simulink model "celBebe"  (R2020a)
settings: Solver=FixedStepAuto  StartTime=0.0  StopTime=10.0  RelTol=1e-3
undefined symbols (not defined in the file): AA, B9, blue, green, red
libraries: androiduilib x4, androidaudiovideolib x3, simulink x2, androidcommunicationlib x1, visionsources x1
settings Model: Creator=luisi  LastModifiedBy=luisi
settings OptimizationCC: EnhancedBackFolding=on  PassReuseOutputArgsAs=Individual arguments  ZeroExternalMemoryAtStartup=off  ZeroInternalMemoryAtStartup=off  MaxStackSize=64  OptimizeBlockOrder=speed  DifferentSizesBufferReuse=on  OptimizationCustomize=off  EfficientTunableParamExpr=on
settings DebuggingCC: ParameterTunabilityLossMsg=error
settings HardwareCC: ProdBitPerPointer=32  ProdBitPerSizeT=32  ProdBitPerPtrDiffT=32  ProdLargestAtomicInteger=Long  ProdLargestAtomicFloat=Double  ProdWordSize=32  ProdHWDeviceType=ARM Compatible->ARM Cortex
settings SFSimCC: MATLABDynamicMemAlloc=off
settings RTWCC: SystemTargetFile=ert.tlc  HardwareBoard=Android Device  TemplateMakefile=ert_default_tmf  RTWVerbose=off  Toolchain=Android SDK/NDK Tools
settings CodeAppCC: ForceParamTrailComments=on  IgnoreCustomStorageClasses=off  OperatorAnnotations=on  SimulinkDataObjDesc=on  SFDataObjDesc=on  InsertBlockDesc=on
settings ERTTargetCC: ExtModeMexArgs='localhost'

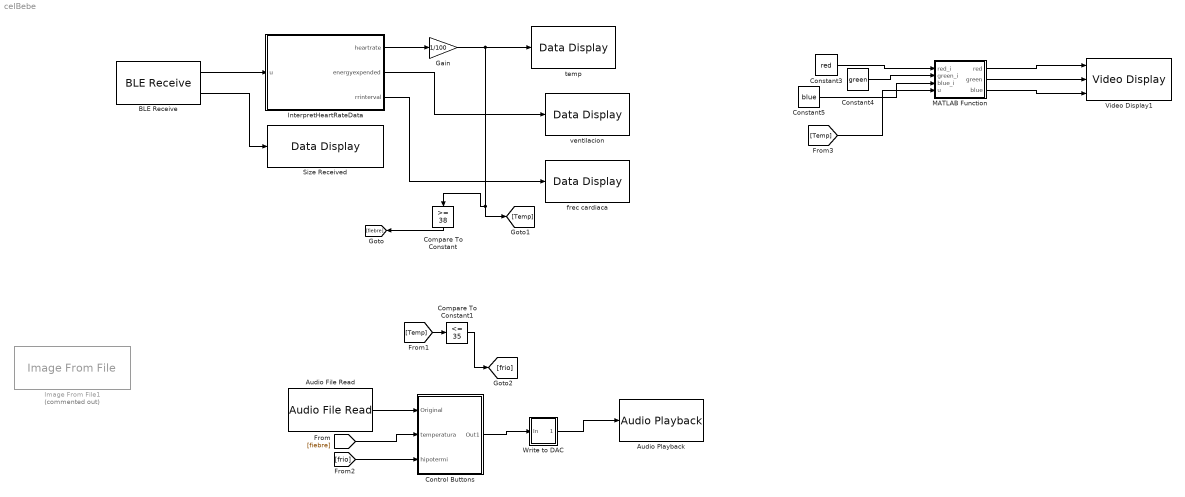
== system celBebe ==
  " BLE Receive" : androidcommunicationlib/BLE Receive  DeviceMode=Central (Client)  BluetoothAddress=4F:B9:1D:3B:34:AA  CharUUID=00002a37-0000-1000-8000-00805f9b34fb  ServiceUUID=0000180d-0000-1000-8000-00805f9b34fb  device=Redmi  character="Heart Rate\\Heart Rate  Measurement"  CustomService=off  ServiceName=Heart Rate  CharacteristicName="Heart Rate  Measurement"  CustomServiceUUID=<Enter Service UUID>  CustomCharUUID=<Enter Characteristic UUID>  DataSize=7  SampleTime=0.1  charseruuid=00001801-0000-1000-8000-00805f9b34fb\00002a05-0000-1000-8000-00805f9b34fb  seruuid=00001810-0000-1000-8000-00805f9b34fb  PeripheralService=0000180d-0000-1000-8000-00805f9b34fb  PeripheralCharacteristic=00002a37-0000-1000-8000-00805f9b34fb  chruuid=00002a37-0000-1000-8000-00805f9b34fb  BLEId=celBebe/_BLE_Receive  Devicename=Redmi  IsCustomService=0
      settings: SourceProductBaseCode=ANDROID
  Audio File Read : androidaudiovideolib/Audio File Read  FileName=C:\Users\luisi\Downloads\baby.mp3  FrameSize=4410
      settings: SourceProductBaseCode=ANDROID
  Audio Playback : androidaudiovideolib/Audio Playback  SampleFreq=44100  AudioSamplingFreq=44100  SampleTime=0.1  DeviceStr=0  QueueDuration=0  BlockPlatform=Android
      settings: SourceProductBaseCode=ANDROID
  Compare To Constant : simulink/Logic and Bit Operations/Compare To Constant  relop=>=  const=38  OutDataTypeStr=boolean
  Compare To Constant1 : simulink/Logic and Bit Operations/Compare To Constant  relop=<=  const=35  OutDataTypeStr=boolean
  Constant3 : Constant  Value=red
  Constant4 : Constant  Value=green
  Constant5 : Constant  Value=blue
  Control Buttons : Subsystem
  Gain : Gain  Gain=1/100
  Image From File1 : visionsources/Image From File  Tag=vipblks_nd  Commented=on  FileName=C:\Users\luisi\Downloads\victoria.jpg  Ts=inf  imagePorts=Separate color signals  OutPortLabels=R|G|B  ImageDataType=uint8  sdImageDataType=uint(8)  Signed=on  WordLength=16  FractionLengthMode=User-defined  FractionLength=15
  InterpretHeartRateData : MATLAB Function  TreatAsAtomicUnit=on
  MATLAB Function : MATLAB Function  TreatAsAtomicUnit=on
  Size Received : androiduilib/Data Display  DataDisplayId=celBebe/Size_Received  Format=Float  Precision=6  SimulateUsing=Code generation  blockPlatform=Android
      settings: SourceProductBaseCode=ANDROID
  Video Display1 : androidaudiovideolib/Video Display  BlockPlatform=Android
      settings: SourceProductBaseCode=ANDROID
  Write to DAC : Subsystem
  frec cardiaca : androiduilib/Data Display  DataDisplayId=celBebe/frec_cardiaca  Format=Integer  Precision=6  SimulateUsing=Code generation  blockPlatform=Android
      settings: SourceProductBaseCode=ANDROID
  temp : androiduilib/Data Display  DataDisplayId=celBebe/temp  Format=Float  Precision=2  SimulateUsing=Code generation  blockPlatform=Android
      settings: SourceProductBaseCode=ANDROID
  ventilacion : androiduilib/Data Display  DataDisplayId=celBebe/ventilacion  Format=Integer  Precision=6  SimulateUsing=Code generation  blockPlatform=Android
      settings: SourceProductBaseCode=ANDROID
  wires:
  " BLE Receive"/2 -> Size Received/1
  " BLE Receive"/1 -> InterpretHeartRateData/1(u)
  Compare To Constant/1 -> [fiebre]
  InterpretHeartRateData/1(heartrate) -> Gain/1
  InterpretHeartRateData/2(energyexpended) -> ventilacion/1
  InterpretHeartRateData/3(rrinterval) -> frec cardiaca/1
  Audio File Read/1 -> Control Buttons/1(Original)
  Write to DAC/1(Out) -> Audio Playback/1
  Control Buttons/1(Out1) -> Write to DAC/1(In)
  [fiebre] -> Control Buttons/2(temperatura)
  Gain/1 -> [Temp], Compare To Constant/1, temp/1
  [Temp] -> Compare To Constant1/1
  Compare To Constant1/1 -> [frio]
  [frio] -> Control Buttons/3(hipotermi)
  Constant4/1 -> MATLAB Function/2(green_i)
  Constant5/1 -> MATLAB Function/3(blue_i)
  MATLAB Function/2(green) -> Video Display1/2
  MATLAB Function/1(red) -> Video Display1/1
  [Temp] -> MATLAB Function/4(u)
  Constant3/1 -> MATLAB Function/1(red_i)
  MATLAB Function/3(blue) -> Video Display1/3

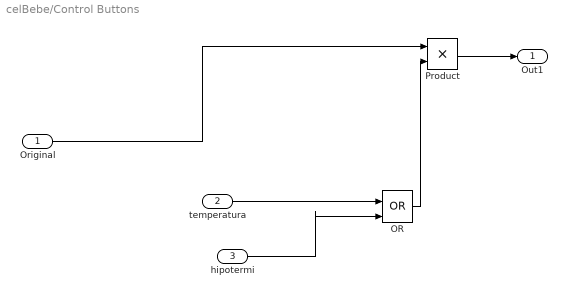
== system celBebe/Control Buttons ==
  Original : Inport
  temperatura : Inport  Port=2
  hipotermi : Inport  Port=3
  OR : Logic  Operator=OR  IconShape=distinctive  AllPortsSameDT=off  OutDataTypeStr=boolean
  Product : Product
  Out1 : Outport  VectorParamsAs1DForOutWhenUnconnected=off
  wires:
  Product/1 -> Out1/1
  Original/1 -> Product/1
  temperatura/1 -> OR/1
  hipotermi/1 -> OR/2
  OR/1 -> Product/2

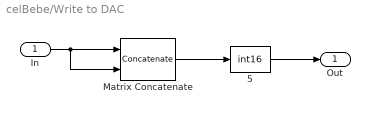
== system celBebe/Write to DAC ==
  In : Inport
  " 5" : DataTypeConversion  OutDataTypeStr=int16
  Matrix Concatenate : Concatenate  Mode=Multidimensional array  ConcatenateDimension=2
  Out : Outport  VectorParamsAs1DForOutWhenUnconnected=off
  wires:
  In/1 -> Matrix Concatenate/2, Matrix Concatenate/1
  Matrix Concatenate/1 -> " 5"/1
  " 5"/1 -> Out/1

== matlab function celBebe/MATLAB Function ==
  data: red_i input; green_i input; red output; green output; blue_i input; u input; blue output
function [red, green, blue] = fcn(red_i, green_i,blue_i,u)
    frio =205;
    fiebre=600;
    if u<37 && u>36 %normal
        blue=blue_i;
        red=red_i;
        green=green_i;
        
    elseif u>38 %fiebre
        
        %cachete izq
        for c= 430:550
            for m=550:700
                red_i(c,m)= fiebre;
            end
        end
        %cachete derecho
        for c= 470:600
            for m=300:400
                red_i(c,m)=fiebre;
                
            end
        end
        %labios
        for c= 550:600
            for m=440:530
                red_i(c,m)=fiebre;
            end
        end
        blue=blue_i;
        red=red_i;
        green=green_i;
    else
        %frio
          %cachete izq
        for c= 430:550
            for m=550:700
                blue_i(c,m)=frio;
                
            end
        end
        %cachete derecho
        for c= 470:600
            for m=300:400
                blue_i(c,m)=frio;
                %redcalor(c,m)=calor;
            end
        end
        %labios
        for c= 550:600
            for m=440:530
                blue_i(c,m)=frio;
                %redcalor(c,m)=380;
            end
        end
        blue=blue_i;
        red=red_i;
        green=green_i;
    end

== matlab function celBebe/InterpretHeartRateData ==
  data: u input; heartrate output; energyexpended output; rrinterval output
function [heartrate, energyexpended, rrinterval ] = InterpretHeartRateData(u)
flag = uint8(u(1));
heartrate = uint16(0);
energyexpended=uint16(0);
rrinterval = uint16(0);
b = bitget(flag,8:-1:1);

 if b(8) == 0
     format = uint8(2);
     heartrate = uint16(u(2));
 else
     format = uint8(3);
     heartrate = typecast([u(2) u(3)], 'uint16');
 end
 
 if b(5) == 1
     energy = uint8(2);
     energyexpended = typecast([u(format +1) u(format + 2)], 'uint16');
 else
     energy = uint8(0);
     energyexpended = uint16(0);
 end
 
 if b(4) == 1
     rrinterval = typecast([u(format +energy + 1) u(format + energy + 2)],'uint16');
 else
     rrinterval = uint16(0);
 end
end
